simulink model "admittance_control"  (R2020b)
settings: Solver=FixedStepAuto  StartTime=0.0  StopTime=10  FixedStep=Ts  RelTol=1e-3
undefined symbols (not defined in the file): dqi, K, KD, KDt, KP, KPt, Mt, myRobot, qi, xf, xi, xr
settings Model: Creator=simon  LastModifiedBy=simon
settings SolverCC: ZeroCrossControl=DisableAll

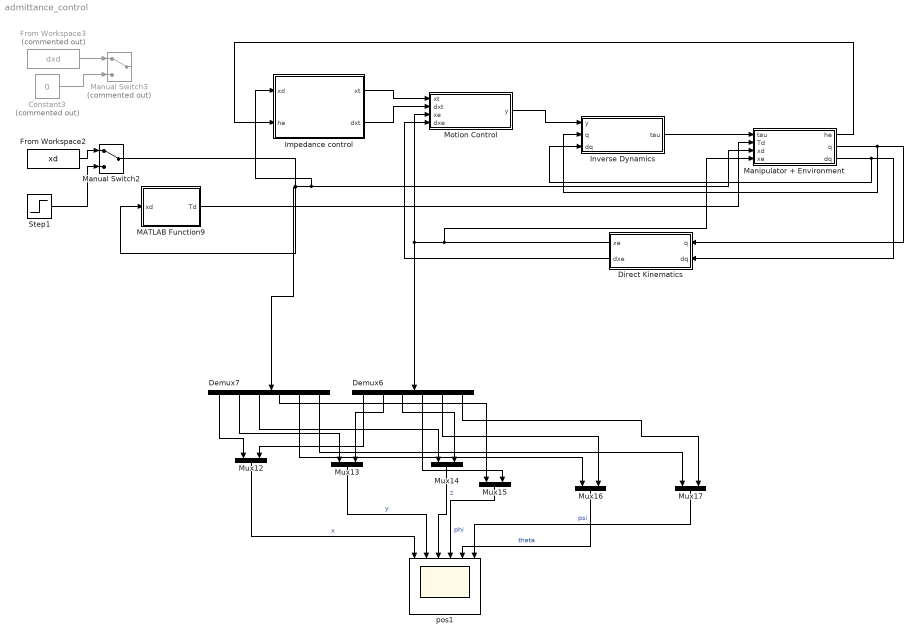
== system admittance_control ==
  Constant3 : Constant  Commented=on  Value=0
  Demux6 : Demux  Outputs=6
  Demux7 : Demux  Outputs=6
  Direct Kinematics : Subsystem
  From Workspace2 : FromWorkspace  VariableName=xd
  From Workspace3 : FromWorkspace  Commented=on  VariableName=dxd
  Impedance control : Subsystem
  Inverse Dynamics : Subsystem
  MATLAB Function9 : MATLAB Function  TreatAsAtomicUnit=on
  Manipulator + Environment : Subsystem
  Manual Switch2 : ManualSwitch
  Manual Switch3 : ManualSwitch  Commented=on
  Motion Control : Subsystem
  Mux{12..17} (6 alike) : Mux  Inputs=2
  Step1 : Step  Before=xi  After=xf  SampleTime=0
  pos1 : Scope  NumInputPorts=6
  wires:
  Inverse Dynamics/1(tau) -> Manipulator + Environment/1(tau)
  Manipulator + Environment/2(q) -> Inverse Dynamics/2(q), Direct Kinematics/1(q)
  Manipulator + Environment/3(dq) -> Inverse Dynamics/3(dq), Direct Kinematics/2(dq)
  Manipulator + Environment/1(he) -> Impedance control/2(he)
  Step1/1 -> Manual Switch2/2
  From Workspace2/1 -> Manual Switch2/1
  From Workspace3/1 -> Manual Switch3/1
  Constant3/1 -> Manual Switch3/2
  MATLAB Function9/1(Td) -> Manipulator + Environment/2(Td)
  Demux7/3 -> Mux14/1
  Direct Kinematics/1(xe) -> Motion Control/3(xe), Demux6/1, Manipulator + Environment/4(xe)
  Mux17/1 -> pos1/6  "psi"
  Demux6/5 -> Mux16/2
  Demux7/6 -> Mux17/1
  Mux16/1 -> pos1/5  "theta"
  Mux15/1 -> pos1/4  "phi"
  Manual Switch2/1 -> Demux7/1, MATLAB Function9/1(xd), Manipulator + Environment/3(xd), Impedance control/1(xd)
  Demux7/4 -> Mux15/1
  Demux7/2 -> Mux13/1
  Demux6/6 -> Mux17/2
  Mux14/1 -> pos1/3  "z"
  Demux7/1 -> Mux12/1
  Demux6/2 -> Mux13/2
  Demux7/5 -> Mux16/1
  Demux6/1 -> Mux12/2
  Demux6/3 -> Mux14/2
  Mux12/1 -> pos1/1  "x"
  Demux6/4 -> Mux15/2
  Mux13/1 -> pos1/2  "y"
  Impedance control/1(xt) -> Motion Control/1(xt)
  Motion Control/1(y) -> Inverse Dynamics/1(y)
  Impedance control/2(dxt) -> Motion Control/2(dxt)
  Direct Kinematics/2(dxe) -> Motion Control/4(dxe)

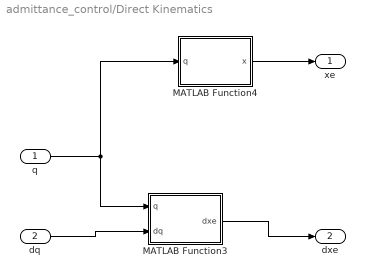
== system admittance_control/Direct Kinematics ==
  q : Inport
  dq : Inport  Port=2
  MATLAB Function3 : MATLAB Function  TreatAsAtomicUnit=on
  MATLAB Function4 : MATLAB Function  TreatAsAtomicUnit=on
  xe : Outport
  dxe : Outport  Port=2
  wires:
  MATLAB Function3/1(dxe) -> dxe/1
  dq/1 -> MATLAB Function3/2(dq)
  q/1 -> MATLAB Function4/1(q), MATLAB Function3/1(q)
  MATLAB Function4/1(x) -> xe/1

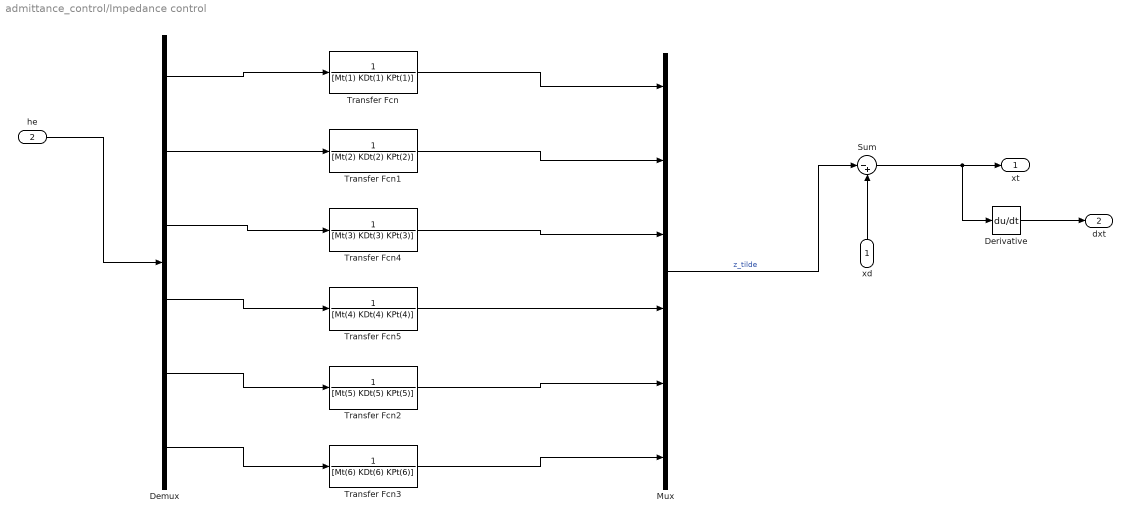
== system admittance_control/Impedance control ==
  xd : Inport
  he : Inport  Port=2
  Demux : Demux  Outputs=6
  Derivative : Derivative
  Mux : Mux  Inputs=6
  Sum : Sum  Inputs=|-+
  Transfer Fcn : TransferFcn  Denominator=[Mt(1) KDt(1) KPt(1)]
  Transfer Fcn1 : TransferFcn  Denominator=[Mt(2) KDt(2) KPt(2)]
  Transfer Fcn2 : TransferFcn  Denominator=[Mt(5) KDt(5) KPt(5)]
  Transfer Fcn3 : TransferFcn  Denominator=[Mt(6) KDt(6) KPt(6)]
  Transfer Fcn4 : TransferFcn  Denominator=[Mt(3) KDt(3) KPt(3)]
  Transfer Fcn5 : TransferFcn  Denominator=[Mt(4) KDt(4) KPt(4)]
  xt : Outport
  dxt : Outport  Port=2
  wires:
  he/1 -> Demux/1
  Mux/1 -> Sum/1  "z_tilde"
  xd/1 -> Sum/2
  Sum/1 -> Derivative/1, xt/1
  Derivative/1 -> dxt/1
  Demux/1 -> Transfer Fcn/1
  Demux/2 -> Transfer Fcn1/1
  Demux/3 -> Transfer Fcn4/1
  Demux/4 -> Transfer Fcn5/1
  Demux/5 -> Transfer Fcn2/1
  Demux/6 -> Transfer Fcn3/1
  Transfer Fcn/1 -> Mux/1
  Transfer Fcn1/1 -> Mux/2
  Transfer Fcn4/1 -> Mux/3
  Transfer Fcn5/1 -> Mux/4
  Transfer Fcn2/1 -> Mux/5
  Transfer Fcn3/1 -> Mux/6

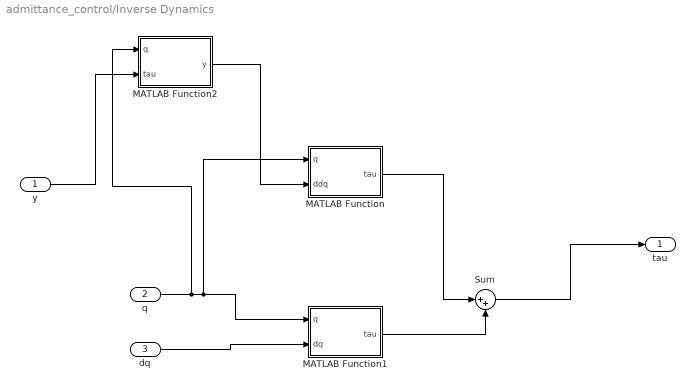
== system admittance_control/Inverse Dynamics ==
  y : Inport
  q : Inport  Port=2
  dq : Inport  Port=3
  MATLAB Function : MATLAB Function  TreatAsAtomicUnit=on
  MATLAB Function1 : MATLAB Function  TreatAsAtomicUnit=on
  MATLAB Function2 : MATLAB Function  TreatAsAtomicUnit=on
  Sum : Sum  Inputs=|++
  tau : Outport
  wires:
  MATLAB Function1/1(tau) -> Sum/2
  MATLAB Function/1(tau) -> Sum/1
  Sum/1 -> tau/1
  dq/1 -> MATLAB Function1/2(dq)
  q/1 -> MATLAB Function2/1(q), MATLAB Function/1(q), MATLAB Function1/1(q)
  y/1 -> MATLAB Function2/2(tau)
  MATLAB Function2/1(y) -> MATLAB Function/2(ddq)

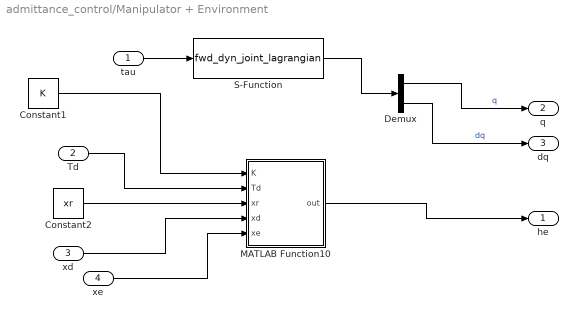
== system admittance_control/Manipulator + Environment ==
  tau : Inport
  Td : Inport  Port=2
  xd : Inport  Port=3
  xe : Inport  Port=4
  Constant1 : Constant  Value=K
  Constant2 : Constant  Value=xr
  Demux : Demux  Outputs=2
  MATLAB Function10 : MATLAB Function  TreatAsAtomicUnit=on
  S-Function : S-Function  FunctionName=fwd_dyn_joint_lagrangian  Parameters=myRobot,qi,dqi  SFunctionDeploymentMode=off  EnableBusSupport=off
  he : Outport
  q : Outport  Port=2
  dq : Outport  Port=3
  wires:
  tau/1 -> S-Function/1
  Constant1/1 -> MATLAB Function10/1(K)
  Constant2/1 -> MATLAB Function10/3(xr)
  Td/1 -> MATLAB Function10/2(Td)
  xd/1 -> MATLAB Function10/4(xd)
  xe/1 -> MATLAB Function10/5(xe)
  S-Function/1 -> Demux/1
  Demux/1 -> q/1  "q"
  Demux/2 -> dq/1  "dq"
  MATLAB Function10/1(out) -> he/1

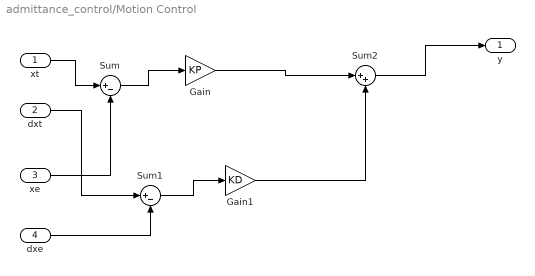
== system admittance_control/Motion Control ==
  xt : Inport
  dxt : Inport  Port=2
  xe : Inport  Port=3
  dxe : Inport  Port=4
  Gain : Gain  Gain=KP
  Gain1 : Gain  Gain=KD
  Sum : Sum  Inputs=|+-
  Sum1 : Sum  Inputs=|+-
  Sum2 : Sum  Inputs=|++
  y : Outport
  wires:
  xt/1 -> Sum/1
  xe/1 -> Sum/2
  Sum/1 -> Gain/1
  dxt/1 -> Sum1/1
  dxe/1 -> Sum1/2
  Sum1/1 -> Gain1/1
  Gain/1 -> Sum2/1
  Gain1/1 -> Sum2/2
  Sum2/1 -> y/1

== matlab function admittance_control/Direct Kinematics/MATLAB Function3 ==
  data: q input; dxe output; dq input
function dxe = Ja(q, dq)

dxe = getJa(q)*dq;

== matlab function admittance_control/Inverse Dynamics/MATLAB Function2 ==
  data: q input; y output; tau input
function y = invJa(q, tau)

y = getInvJa(q)*tau;

== matlab function admittance_control/Direct Kinematics/MATLAB Function4 ==
  data: q input; x output
function x = k(q)

x = getK(q);

== matlab function admittance_control/Inverse Dynamics/MATLAB Function ==
  data: q input size=3; tau output; ddq input size=3
function tau = B(q, ddq)

tau = getB(q)*ddq;

== matlab function admittance_control/Inverse Dynamics/MATLAB Function1 ==
  data: q input size=3; tau output; dq input size=3
function tau = n(q, dq)

tau = getN(q, dq);

== matlab function admittance_control/Manipulator + Environment/MATLAB Function10 ==
  data: K input; Td input; out output size=6; xr input; xd input; xe input size=6
function out = hde(K,Td, xr, xd, xe)
%consider the interaction only in z direction
if xe(3) < xr(3)
    dxrd = xd-xr;
    dxed = xd-xe;
    dxre = dxrd-dxed;
    he = K*dxre;
else
    he = zeros(6,1);
end

out = he;

== matlab function admittance_control/MATLAB Function9 ==
  data: xd input; Td output
function Td = getTd(xd)
Rd = eul2rotm(xd(4:6)','ZYZ');
t = xd(1:3);
Td = [Rd t
    zeros(1,3) 1];
